simulink model "planner_contral"  (R2023b)
settings: Solver=FixedStepAuto  StartTime=0  StopTime=inf  FixedStep=0.001  RelTol=1e-3
undefined symbols (not defined in the file): aubr, c_factor, cf, cr, iniObsHeading1, iniObsHeading2, iniObsPos1, iniObsPos2, KD_PID_distance, KD_PID_speed, KI_PID_distance, KI_PID_speed, KP_PID_distance, KP_PID_speed, la, lb, LQR_K1, LQR_K2, LQR_K3, LQR_K4, m, rack_displacement, refInfo_obs1, refInfo_obs2, right_wheel_ground, rightWaypoints, tablebr, vubr, vx_break_point
libraries: Solver_SF x1
(part 6 of 8)

== matlab function planner_contral/decision_planning/EMplanner/spee planning with quadratic programming (qp) ==
  data: plan_start_s_dot input; qp_s_init output; plan_start_s_dot2 input; dp_speed_s input; dp_speed_t input; s_lb input; s_ub input; s_dot_lb input; s_dot_ub input; qp_s_dot_init output; qp_s_dot2_init output; relative_time_init output; w_cost_s_dot2 input; w_cost_v_ref input; w_cost_jerk input; w_ref_s input; speed_reference input
function [qp_s_init,qp_s_dot_init,qp_s_dot2_init,relative_time_init] = fcn(plan_start_s_dot,...
    plan_start_s_dot2,dp_speed_s,dp_speed_t,s_lb,s_ub,s_dot_lb,s_dot_ub,w_cost_s_dot2,w_cost_v_ref,w_cost_jerk,w_ref_s,speed_reference)

% 融合有限松弛约束的 QP 速度优化
% 原变量：每个节点 [s, s_dot, s_dot2]
% 新增变量：每个非起点节点 eps_s，用于轻微放松 s_lb / s_ub
%
% 松弛形式：
%   s >= s_lb - eps_s
%   s <= s_ub + eps_s
%   0 <= eps_s <= eps_s_max
%
% 注意：eps_s 惩罚权重较大，因此只有在原始边界接近不可行时才会启用

coder.extrinsic("solve_quadprog_safe");

% ---------- 参数 ----------
n = 17;
max_qp_node = 17;
default_speed_ub = 30;
large_s_bound = 1e4;

% 松弛变量参数
eps_s_max = 0.5;      % 最大允许纵向边界松弛量，单位 m
w_slack_s = 1e4;      % 松弛变量惩罚权重，越大越不愿意使用松弛

% ---------- 输出初始化 ----------
qp_s_init = ones(n,1) * nan;
qp_s_dot_init = ones(n,1) * nan;
qp_s_dot2_init = ones(n,1) * nan;
relative_time_init = ones(n,1) * nan;

% ---------- 计算有效 DP 点数 ----------
dp_speed_end = 16;
for i = 1:length(dp_speed_s)
    if isnan(dp_speed_s(i))
        dp_speed_end = i - 1;
        break;
    end
end

% DP 无有效点时，直接保守输出起点
if dp_speed_end < 1
    qp_s_init(1) = 0;
    qp_s_dot_init(1) = plan_start_s_dot;
    qp_s_dot2_init(1) = plan_start_s_dot2;
    relative_time_init(1) = 0;
    return;
end

recommend_T = dp_speed_t(dp_speed_end);
if ~isfinite(recommend_T) || recommend_T <= 0
    recommend_T = 8.0;
end

qp_size = dp_speed_end + 1;
if qp_size > max_qp_node
    qp_size = max_qp_node;
    dp_speed_end = qp_size - 1;
end

dt = recommend_T / dp_speed_end;
if ~isfinite(dt) || dt <= 0
    dt = 0.5;
end

% 原始变量数量：[s, v, a] * qp_size
old_var_num = 3 * qp_size;

% 新增松弛变量数量：非起点节点 qp_size - 1
slack_num = qp_size - 1;

% 总变量数量
var_num = old_var_num + slack_num;

% eps_s 在 X 中的起始位置
eps_offset = old_var_num;

% ---------- 等式约束：运动学连续性 ----------
% 原形式仍然是 Aeq' * X == beq
Aeq = zeros(var_num, 2*qp_size - 2);
beq = zeros(2*qp_size - 2, 1);

A_sub = [1, 0;
         dt, 1;
         (1/3)*dt^2, (1/2)*dt;
         -1, 0;
         0, -1;
         (1/6)*dt^2, dt/2];

for i = 1:qp_size - 1
    Aeq(3*i-2:3*i+3, 2*i-1:2*i) = A_sub;
end

% ---------- 不等式约束 ----------
% 1. 不允许倒车：s_i - s_{i+1} <= 0
% 2. 松弛下边界：-s_i - eps_i <= -s_lb
% 3. 松弛上边界： s_i - eps_i <=  s_ub

ineq_num = (qp_size - 1) + 2 * (qp_size - 1);
A = zeros(ineq_num, var_num);
b = zeros(ineq_num, 1);

row = 0;

% 不允许 s 后退
for i = 1:qp_size - 1
    row = row + 1;
    A(row, 3*i - 2) = 1;
    A(row, 3*i + 1) = -1;
    b(row) = 0;
end

% s 边界松弛约束
for i = 2:qp_size
    s_idx = 3*i - 2;
    eps_idx = eps_offset + (i - 1);

    cur_lb = s_lb(i-1);
    cur_ub = s_ub(i-1);

    % 防止 NaN / Inf 进入 quadprog
    if ~isfinite(cur_lb)
        cur_lb = 0;
    end

    if ~isfinite(cur_ub)
        cur_ub = large_s_bound;
    end

    cur_lb = max(cur_lb, 0);

    if cur_ub <= cur_lb
        cur_ub = cur_lb + 0.5;
    end

    % s_i >= cur_lb - eps_i
    % 等价于 -s_i - eps_i <= -cur_lb
    row = row + 1;
    A(row, s_idx) = -1;
    A(row, eps_idx) = -1;
    b(row) = -cur_lb;

    % s_i <= cur_ub + eps_i
    % 等价于 s_i - eps_i <= cur_ub
    row = row + 1;
    A(row, s_idx) = 1;
    A(row, eps_idx) = -1;
    b(row) = cur_ub;
end

% ---------- 变量上下界 ----------
lb = -inf(var_num, 1);
ub = inf(var_num, 1);

% 起点硬约束
lb(1) = 0;
lb(2) = plan_start_s_dot;
lb(3) = plan_start_s_dot2;
ub(1) = lb(1);
ub(2) = lb(2);
ub(3) = lb(3);

% 非起点的速度、加速度约束
for i = 2:qp_size
    s_idx = 3*i - 2;
    v_idx = 3*i - 1;
    a_idx = 3*i;

    % s 的具体上下边界已经通过 A,b 加入，这里只给物理范围
    lb(s_idx) = 0;
    ub(s_idx) = large_s_bound;

    cur_v_lb = s_dot_lb(i-1);
    cur_v_ub = s_dot_ub(i-1);

    if ~isfinite(cur_v_lb)
        cur_v_lb = 0;
    end

    if ~isfinite(cur_v_ub)
        cur_v_ub = default_speed_ub;
    end

    cur_v_lb = max(cur_v_lb, 0);

    if cur_v_ub <= cur_v_lb
        cur_v_ub = cur_v_lb + 0.1;
    end

    lb(v_idx) = cur_v_lb;
    ub(v_idx) = cur_v_ub;

    % 加速度硬约束
    lb(a_idx) = -6;
    ub(a_idx) = 4;
end

% 松弛变量约束：0 <= eps_s <= eps_s_max
for i = 1:slack_num
    eps_idx = eps_offset + i;
    lb(eps_idx) = 0;
    ub(eps_idx) = eps_s_max;
end

% ---------- 构造目标函数 ----------
A_s_dot2 = zeros(old_var_num, old_var_num);
A_jerk = zeros(old_var_num, qp_size - 1);
A_ref = zeros(old_var_num, old_var_num);
A_ref_s = zeros(old_var_num, old_var_num);

A4_sub = [0; 0; 1; 0; 0; -1];

for i = 1:qp_size
    A_s_dot2(3*i, 3*i) = 1;
    A_ref(3*i-1, 3*i-1) = 1;
    A_ref_s(3*i-2, 3*i-2) = 1;
end

for i = 1:qp_size - 1
    A_jerk(3*i-2:3*i+3, i) = A4_sub;
end

H_old = w_cost_s_dot2 * (A_s_dot2 * A_s_dot2') ...
      + w_cost_jerk * (A_jerk * A_jerk') ...
      + w_cost_v_ref * (A_ref * A_ref') ...
      + w_ref_s * (A_ref_s * A_ref_s');

H_old = 2 * H_old;

H = zeros(var_num, var_num);
H(1:old_var_num, 1:old_var_num) = H_old;

% 松弛变量二次惩罚
for i = 1:slack_num
    eps_idx = eps_offset + i;
    H(eps_idx, eps_idx) = 2 * w_slack_s;
end

f = zeros(var_num, 1);

% 推荐速度代价
for i = 1:qp_size
    f(3*i-1) = -2 * w_cost_v_ref * speed_reference;
end

% DP 纵向位置参考代价
for i = 1:dp_speed_end
    f(3*i-2) = -2 * w_ref_s * dp_speed_s(i);
end

% ---------- 求解 QP ----------
X = zeros(var_num, 1);
qp_ok = false;

[X, qp_ok] = solve_quadprog_safe(H, f, A, b, Aeq', beq, lb, ub, var_num);



if ~qp_ok
    qp_s_init(1) = 0;
    qp_s_dot_init(1) = plan_start_s_dot;
    qp_s_dot2_init(1) = plan_start_s_dot2;
    relative_time_init(1) = 0;

    last_s = 0;
    last_v = plan_start_s_dot;

    for i = 2:qp_size
        cur_s = dp_speed_s(i-1);

        if ~isfinite(cur_s)
            cur_s = last_s + max(last_v, 0) * dt;
        end

        cur_s = max(cur_s, last_s);

        if i >= 3
            cur_v = (cur_s - last_s) / dt;
        else
            cur_v = plan_start_s_dot;
        end

        if ~isfinite(cur_v)
            cur_v = speed_reference;
        end

        cur_v = max(cur_v, 0);
        cur_v = min(cur_v, default_speed_ub);

        qp_s_init(i) = cur_s;
        qp_s_dot_init(i) = cur_v;
        qp_s_dot2_init(i) = 0;
        relative_time_init(i) = (i - 1) * dt;

        last_s = cur_s;
        last_v = cur_v;
    end

    return;
end

% ---------- 正常输出 ----------
for i = 1:qp_size
    qp_s_init(i) = X(3*i - 2);
    qp_s_dot_init(i) = X(3*i - 1);
    qp_s_dot2_init(i) = X(3*i);
    relative_time_init(i) = (i - 1) * dt;
end

end

== matlab function planner_contral/decision_planning/EMplanner/Cartesian2Frenet/MATLAB Function2 ==
  data: ax_set input; s_dot2_set output; ay_set input; proj_heading_set input; proj_kappa_set input; l_set input; s_dot_set input; dl_set input; l_dot2_set output; ddl_set output
function [s_dot2_set,l_dot2_set,ddl_set] = fcn(ax_set,ay_set,proj_heading_set,proj_kappa_set,l_set,s_dot_set,dl_set)
%由于不知道有多少个点需要做坐标转换，设一个最大值做缓冲
n = 128;
% 输出初始化
s_dot2_set = ones(n,1)*nan;
l_dot2_set = ones(n,1)*nan;
ddl_set = ones(n,1)*nan;

for i = 1:length(l_set)
    if isnan(l_set(i))
       break;
    end
    a_h = [ax_set(i);ay_set(i)];
    n_r = [-sin(proj_heading_set(i));cos(proj_heading_set(i))];
    t_r = [cos(proj_heading_set(i));sin(proj_heading_set(i))];
    %近似认为dkr/ds 为0 简化计算
    l_dot2_set(i) = a_h'*n_r - proj_kappa_set(i) * (1 - proj_kappa_set(i) * l_set(i)) * s_dot_set(i)^2;
    s_dot2_set(i) = (1/(1 - proj_kappa_set(i) * l_set(i)))* (a_h' * t_r + 2 * proj_kappa_set(i) * dl_set(i) * s_dot_set(i)^2);
    % 要考虑加速度为0的情况
    if (s_dot2_set(i) < 1e-6)
        ddl_set(i) = 0;
    else
        ddl_set(i) = (l_dot2_set(i) - dl_set(i)*s_dot2_set(i))/(s_dot_set(i)^2);
    end
end

== matlab function planner_contral/decision_planning/EMplanner/generate st graph ==
  data: static_obs_s input; static_obs_l input; static_obs_heading input; dynamic_obs_s_set input; dynamic_obs_l_set input; dynamic_obs_heaidng_set input; static_obs_st_s_lb_set output; tra_s input; tra_l input; tra_path_indexs input; static_obs_st_s_ub_set output; dynamic_obs_st_s_lb_set output; dynamic_obs_st_s_ub_set output; obs_st_t_lb_set output; obs_st_t_ub_set output; static_obs_st_t_lb_set output; static_obs_st_t_ub_set output; plan_s_dot input; plan_l input; plan_s input; dynamic_obs_s_dot input; dynamic_obs_st_t_lb_set output; dynamic_obs_st_t_ub_set output
%%
% ============================================================
% generate ST graph
% 改进点：
% 1) 静态障碍物在整个规划时域内生成固定 ST 占用带；
% 2) 动态障碍物按 obs_s_dot 在每个时间步预测位置，生成连续 ST 占用带；
% 3) 多个障碍物暂时采用保守合并：同一时刻取最小 lb 和最大 ub；
% 4) 输入输出接口保持不变，便于直接替换原 Simulink MATLAB Function。
% ============================================================
function [static_obs_st_s_lb_set, static_obs_st_s_ub_set, ...
          dynamic_obs_st_s_lb_set, dynamic_obs_st_s_ub_set, ...
          obs_st_t_lb_set, obs_st_t_ub_set, ...
          static_obs_st_t_lb_set, static_obs_st_t_ub_set, ...
          dynamic_obs_st_t_lb_set, dynamic_obs_st_t_ub_set] = ...
    fcn(static_obs_s, static_obs_l, static_obs_heading, ...
        dynamic_obs_s_set, dynamic_obs_l_set, dynamic_obs_heaidng_set, ...
        tra_s, tra_l, tra_path_indexs, ...
        plan_s_dot, plan_l, plan_s, dynamic_obs_s_dot)

% -------- 基本参数 --------
n  = 81;
dt = 0.1;
t_grid = (0:dt:8)';

% -------- 初始化输出 --------
static_obs_st_s_lb_set  = ones(n,1) * inf;
static_obs_st_s_ub_set  = ones(n,1) * -inf;
dynamic_obs_st_s_lb_set = ones(n,1) * inf;
dynamic_obs_st_s_ub_set = ones(n,1) * -inf;

static_obs_st_t_lb_set  = t_grid;
static_obs_st_t_ub_set  = t_grid;
dynamic_obs_st_t_lb_set = t_grid;
dynamic_obs_st_t_ub_set = t_grid;

obs_st_t_lb_set = t_grid;
obs_st_t_ub_set = t_grid;

% -------- 静态障碍物 ST 边界 --------
[static_lb, static_ub] = getStaticBoundFullHorizon( ...
    static_obs_s, static_obs_l, static_obs_heading, ...
    tra_s, tra_l, tra_path_indexs, n, dt, plan_l, plan_s);

static_obs_st_s_lb_set = static_lb;
static_obs_st_s_ub_set = static_ub;

% -------- 动态障碍物 ST 边界 --------
[dynamic_lb, dynamic_ub] = getDynamicBoundFullHorizon( ...
    dynamic_obs_s_set, dynamic_obs_l_set, dynamic_obs_heaidng_set, ...
    tra_s, tra_l, tra_path_indexs, n, dt, plan_l, plan_s, dynamic_obs_s_dot);

dynamic_obs_st_s_lb_set = dynamic_lb;
dynamic_obs_st_s_ub_set = dynamic_ub;

end

%%
% ============================================================
% 静态障碍物：整个规划时域内保持固定 s/l/heading
% ============================================================
function [static_obs_lb, static_obs_ub] = getStaticBoundFullHorizon( ...
    static_obs_s, static_obs_l, static_obs_heading, ...
    tra_s, tra_l, index2s, n, dt, plan_l, plan_s)

vehLength = 5;
vehWidth  = 2;
vehHalfWidth = vehWidth / 2;

latThreshold = 2.7;

safeFront = 0;
safeRear  = 0;

startIgnoreDist = 3.0;

static_obs_lb = ones(n,1) * inf;
static_obs_ub = ones(n,1) * -inf;

% 当前接口只输出一组静态障碍物边界，
% 因此先选择当前规划路径上最近的一个前方障碍物。
best_lb = inf;
best_ub = -inf;
found = false;

for i = 1:length(static_obs_s)

    if isnan(static_obs_s(i))
        break;
    end

    rear_s = static_obs_s(i);
    rear_l = static_obs_l(i);
    heading = static_obs_heading(i);


    egoWidth = 2.0;
    latSafe = 0.2;
    lonSafe = 0.5;

    if ~isObstacleOverlapPathCorridor(rear_s, rear_l, heading, ...
        tra_s, tra_l, vehLength, vehWidth, egoWidth, latSafe, lonSafe)
        continue;
    end

    [lb_temp, ub_temp, valid] = calcObstacleSBound( ...
        rear_s, rear_l, heading, ...
        vehLength, vehHalfWidth, ...
        tra_s, tra_l, index2s);

    if ~valid
        continue;
    end

    lb_temp = lb_temp - safeRear;
    ub_temp = ub_temp + safeFront;

    % 忽略明显在起点附近或后方的障碍物
    if ub_temp <= plan_s + startIgnoreDist
        continue;
    end

    if lb_temp < plan_s + startIgnoreDist
        lb_temp = plan_s + startIgnoreDist;
    end

    % 只选择最近的前方障碍物
    if lb_temp < best_lb
        best_lb = lb_temp;
        best_ub = ub_temp;
        found = true;
    end
end

if found
    for j = 1:n
        static_obs_lb(j) = best_lb;
        static_obs_ub(j) = best_ub;
    end
end

end

%%
% ============================================================
% 动态障碍物：每个时间步用 s = s0 + v*t 预测
% ============================================================
function [dynamic_obs_lb, dynamic_obs_ub] = getDynamicBoundFullHorizon( ...
    dynamic_obs_s, dynamic_obs_l, dynamic_obs_heading, ...
    tra_s, tra_l, index2s, n, dt, plan_l, plan_s, obs_s_dot)

vehLength = 5;
vehWidth  = 2;
vehHalfWidth = vehWidth / 2;

latThreshold = 2.7;

safeFront = 0;
safeRear  = 0;

startIgnoreDist = 3.0;

dynamic_obs_lb = ones(n,1) * inf;
dynamic_obs_ub = ones(n,1) * -inf;

for j = 1:n

    t = (j-1) * dt;

    best_lb = inf;
    best_ub = -inf;
    found = false;

    for i = 1:length(dynamic_obs_s)

        if isnan(dynamic_obs_s(i))
            break;
        end

        s0 = dynamic_obs_s(i);
        l0 = dynamic_obs_l(i);
        heading = dynamic_obs_heading(i);

        if length(obs_s_dot) >= i
            v_obs = obs_s_dot(i);
        else
            v_obs = 0;
        end

        rear_s = s0 + v_obs * t;
        rear_l = l0;
     
        egoWidth = 2.0;
        latSafe = 0.2;
        lonSafe = 0.5;

        if ~isObstacleOverlapPathCorridor(rear_s, rear_l, heading, ...
                tra_s, tra_l, vehLength, vehWidth, egoWidth, latSafe, lonSafe)
           continue;
        end

        [lb_temp, ub_temp, valid] = calcObstacleSBound( ...
            rear_s, rear_l, heading, ...
            vehLength, vehHalfWidth, ...
            tra_s, tra_l, index2s);

        if ~valid
            continue;
        end

        lb_temp = lb_temp - safeRear;
        ub_temp = ub_temp + safeFront;

        if ub_temp <= plan_s + startIgnoreDist
            continue;
        end

        if lb_temp < plan_s + startIgnoreDist
            lb_temp = plan_s + startIgnoreDist;
        end

        % 每个时间步只选择最近的前方动态障碍物
        if lb_temp < best_lb
            best_lb = lb_temp;
            best_ub = ub_temp;
            found = true;
        end
    end

    if found
        dynamic_obs_lb(j) = best_lb;
        dynamic_obs_ub(j) = best_ub;
    end
end

end

%%
% ============================================================
% 根据障碍物 rear_s/rear_l/heading 计算其在参考路径上的 s 占用范围
% ============================================================
function [s_lb, s_ub, valid] = calcObstacleSBound( ...
    rear_s, rear_l, heading, ...
    vehLength, vehHalfWidth, ...
    tra_s, tra_l, index2s)

valid = false;
s_lb = inf;
s_ub = -inf;

% 前端点
front_s = rear_s + vehLength * cos(heading);
front_l = rear_l + vehLength * sin(heading);

% 四个角点
VehPoints = zeros(4,2);

VehPoints(1,1) = rear_s  - vehHalfWidth * sin(heading);
VehPoints(1,2) = rear_l  + vehHalfWidth * cos(heading);

VehPoints(2,1) = front_s - vehHalfWidth * sin(heading);
VehPoints(2,2) = front_l + vehHalfWidth * cos(heading);

VehPoints(3,1) = front_s + vehHalfWidth * sin(heading);
VehPoints(3,2) = front_l - vehHalfWidth * cos(heading);

VehPoints(4,1) = rear_s  + vehHalfWidth * sin(heading);
VehPoints(4,2) = rear_l  - vehHalfWidth * cos(heading);

index_matrix = zeros(4,1);

for z = 1:4

    dist_min = inf;
    index_min = 0;

    for k = 1:length(tra_s)

        if isnan(tra_s(k))
            break;
        end

        dist_s = tra_s(k) - VehPoints(z,1);
        dist_l = tra_l(k) - VehPoints(z,2);
        dist_temp = sqrt(dist_s^2 + dist_l^2);

        if dist_temp < dist_min
            dist_min = dist_temp;
            index_min = k;
        end
    end

    if index_min <= 0
        return;
    end

    index_matrix(z) = index_min;
end

min_index = min(index_matrix);
max_index = max(index_matrix);

if min_index <= 0 || max_index <= 0
    return;
end

if min_index > length(index2s) || max_index > length(index2s)
    return;
end

s_lb = index2s(min_index);
s_ub = index2s(max_index);

if ~isfinite(s_lb) || ~isfinite(s_ub)
    return;
end

if s_ub < s_lb
    temp = s_lb;
    s_lb = s_ub;
    s_ub = temp;
end

valid = true;

end

%%
% 判断障碍物矩形是否与当前规划路径走廊重叠
% rear_s, rear_l: 障碍物后轴/后端中心在 Frenet-like 坐标下的位置
% heading: 障碍物相对于 s-l 坐标的航向角
% tra_s, tra_l: 路径规划 DP+QP 后的最终路径
% obsLength, obsWidth: 障碍物长度和宽度
% egoWidth: ego 车辆宽度
% latSafe: 横向安全裕度
% lonSafe: 纵向安全裕度
function is_conflict = isObstacleOverlapPathCorridor( ...
    rear_s, rear_l, heading, ...
    tra_s, tra_l, obsLength, obsWidth, egoWidth, latSafe, lonSafe)

is_conflict = false;

obsHalfWidth = obsWidth / 2;
egoHalfWidth = egoWidth / 2;

% 横向膨胀后的半宽：障碍物半宽 + ego 半宽 + 安全裕度
latBound = obsHalfWidth + egoHalfWidth + latSafe;

% 纵向膨胀范围
u_min = -lonSafe;
u_max = obsLength + lonSafe;

% 只检查障碍物附近的路径点，避免远处路径点干扰
s_min_check = rear_s - lonSafe - 2.0;
s_max_check = rear_s + obsLength + lonSafe + 2.0;

cos_h = cos(heading);
sin_h = sin(heading);

for k = 1:length(tra_s)

    if isnan(tra_s(k))
        break;
    end

    s_path = tra_s(k);
    l_path = tra_l(k);

    if s_path < s_min_check || s_path > s_max_check
        continue;
    end

    % 将路径点转换到障碍物局部坐标系
    ds = s_path - rear_s;
    dl = l_path - rear_l;

    % u: 沿障碍物车身方向
    % v: 垂直障碍物车身方向
    u =  ds * cos_h + dl * sin_h;
    v = -ds * sin_h + dl * cos_h;

    % 路径中心线进入“障碍物膨胀矩形”，则认为有冲突
    if u >= u_min && u <= u_max && abs(v) <= latBound
        is_conflict = true;
        return;
    end
end

end

== matlab function planner_contral/decision_planning/EMplanner/speed decision with dynamic planning(dp) ==
  data: static_obs_s_lb input; dp_speed_s output; static_obs_s_ub input; dynamic_obs_s_lb input; dynamic_obs_s_ub input; obs_st_t_lb input; obs_st_t_ub input; dp_speed_t output; reference_speed_unlimit input; w_cost_ref_speed input; w_cost_accel input; w_cost_obs input; plan_start_s_dot input
function [dp_speed_s,dp_speed_t] = fcn(static_obs_s_lb,static_obs_s_ub,dynamic_obs_s_lb,dynamic_obs_s_ub,obs_st_t_lb,obs_st_t_ub,reference_speed_unlimit...
    ,w_cost_ref_speed,w_cost_accel,w_cost_obs,plan_start_s_dot)
% 速度动态规划
% 时间从0到8开始规划，最多8秒
% s的范围从0开始到路径规划的path的总长度为止
% 为了减少算力 采用非均匀采样，s越小的越密，越大的越稀疏

s_list = [0:0.5:4.5,...
          5.5:1:14.5,...
          16:1.5:29.5,...
          32:2.5:54.5];
% t 采用均匀采样每 0.5s采样一个点
t_list = 0.5:0.5:8;
% 声明st代价矩阵，表示从起点开始到(i,j)点的最小代价为dp_st_cost(i,j)
% s 采样40个 t 采样 16个 一共是 40 * 16
dp_st_cost = ones(40,16) * inf; % 首先初始化为无穷大
% dp_st_s_dot，表示从起点开始到(i,j)点的最优路径的末速度
dp_st_s_dot = zeros(40,16);
% 需要一个矩阵保持最优路径的前一个节点方便回溯
% dp_st_node(i,j) 表示位置为(i,j)的节点中，最优的上一层节点的行号为dp_st_node(i,j)
dp_st_node = zeros(40,16);
% 计算从dp起点到第一列的cost
for i = 1:length(s_list)
    dp_st_cost(i,1) = CalcDpCost(0,0,i,1,static_obs_s_lb,static_obs_s_ub,obs_st_t_lb,obs_st_t_ub,...
    w_cost_ref_speed,reference_speed_unlimit,w_cost_accel,w_cost_obs,plan_start_s_dot,s_list,t_list,dp_st_s_dot)+...
     CalcDpCost(0,0,i,1,dynamic_obs_s_lb,dynamic_obs_s_ub,obs_st_t_lb,obs_st_t_ub,...
    w_cost_ref_speed,reference_speed_unlimit,w_cost_accel,w_cost_obs,plan_start_s_dot,s_list,t_list,dp_st_s_dot);
    % 计算第一列所有节点的的s_dot，并存储到dp_st_s_dot中
    % 第一列的前一个节点只有起点，起点的s t 都是0
    [s_end,t_end] = CalcSTCoordinate(i,1,s_list,t_list);
    dp_st_s_dot(i,1) = s_end / t_end;
end
% 动态规划主程序
for i = 2:length(t_list)
    % i 为列循环
    for j = 1:length(s_list)
        % j 为行循环
        % 当前行为 j 列为 i
        cur_row = j;
        cur_col = i;
        % 遍历前一列
        for k = 1:length(s_list)
            pre_row = k;
            pre_col = i - 1;
            % 计算边的代价 其中起点为pre_row,pre_col 终点为cur_row cur_col
            cost_temp = CalcDpCost(pre_row,pre_col,cur_row,cur_col,static_obs_s_lb,static_obs_s_ub,obs_st_t_lb,obs_st_t_ub,...
                w_cost_ref_speed,reference_speed_unlimit,w_cost_accel,w_cost_obs,...
                plan_start_s_dot,s_list,t_list,dp_st_s_dot)+ CalcDpCost(pre_row,pre_col,cur_row,cur_col,dynamic_obs_s_lb,dynamic_obs_s_ub,obs_st_t_lb,obs_st_t_ub,...
              w_cost_ref_speed,reference_speed_unlimit,w_cost_accel,w_cost_obs,...
                plan_start_s_dot,s_list,t_list,dp_st_s_dot);
            if cost_temp + dp_st_cost(pre_row,pre_col) < dp_st_cost(cur_row,cur_col)
                dp_st_cost(cur_row,cur_col) = cost_temp + dp_st_cost(pre_row,pre_col);
                % 计算最优的s_dot
                [s_start,t_start] = CalcSTCoordinate(pre_row,pre_col,s_list,t_list);
                [s_end,t_end] = CalcSTCoordinate(cur_row,cur_col,s_list,t_list);
                dp_st_s_dot(cur_row,cur_col) = (s_end - s_start) / (t_end - t_start);
                % 将最短路径的前一个节点的行号记录下来
                dp_st_node(cur_row,cur_col) = pre_row;
            end      
        end
    end
end
% 输出初始化
dp_speed_s = ones(length(t_list),1) * nan;
dp_speed_t = dp_speed_s;
% 找到dp_node_cost 上边界和右边界代价最小的节点
min_cost = inf;
min_row = inf;
min_col = inf;
for i = 1:length(s_list)
    % 遍历右边界
    if dp_st_cost(i,length(t_list)) <= min_cost
        min_cost = dp_st_cost(i,length(t_list));
        min_row = i;
        min_col = length(t_list);
    end
end

for j = 1:length(t_list)
    % 遍历上边界
    if dp_st_cost(1,j) <= min_cost
        min_cost = dp_st_cost(1,j);
        min_row = 1;
        min_col = j;
    end
end
% 这里要注意，虽然我们在t上每0.5s采样一个时间，采了16个点，但是min_col 未必等于16
% 也就是说动态规划的最优解的时间未必是8秒
% 所以我们动态规划最后的输出s t 不一定是写满
% 先把终点的ST输出出来
[dp_speed_s(min_col),dp_speed_t(min_col)] = CalcSTCoordinate(min_row,min_col,s_list,t_list);
% 反向回溯
while min_col ~= 1
    pre_row = dp_st_node(min_row,min_col);
    pre_col = min_col - 1;
    [dp_speed_s(pre_col),dp_speed_t(pre_col)] = CalcSTCoordinate(pre_row,pre_col,s_list,t_list);
    min_row = pre_row;
    min_col = pre_col;
end


end

function cost = CalcDpCost(row_start,col_start,row_end,col_end,obs_st_s_in_set,obs_st_s_out_set,obs_st_t_in_set,obs_st_t_out_set,...
    w_cost_ref_speed,reference_speed,w_cost_accel,w_cost_obs,plan_start_s_dot,s_list,t_list,dp_st_s_dot)
    % 该函数将计算链接两个节点之间边的代价
    % 输入：边的起点的行列号row_start,col_start 边的终点行列号row_end,col_end
          % 障碍物st信息obs_st_s_in_set,obs_st_s_out_set,obs_st_t_in_set,obs_st_t_out_set
          % 推荐速度代价权重w_cost_ref_speed,加速度代价权重w_cost_accel,障碍物代价权重w_cost_obs
          % 推荐速度reference_speed
          % 拼接起点的速度plan_start_s_dot
          % s_list,t_list 采样距离
          % dp_st_s_dot 用于计算加速度
    % 首先计算终点的st坐标
    [s_end,t_end] = CalcSTCoordinate(row_end,col_end,s_list,t_list);
    % 规定起点的行列号为0 
    if row_start == 0
        % 边的起点为dp的起点
        s_start = 0;
        t_start = 0;
        s_dot_start = plan_start_s_dot;
    else
        % 边的起点不是dp的起点
        [s_start,t_start] = CalcSTCoordinate(row_start,col_start,s_list,t_list);
        s_dot_start = dp_st_s_dot(row_start,col_start);
    end
    cur_s_dot = (s_end - s_start) / (t_end - t_start);
    cur_s_dot2 = (cur_s_dot - s_dot_start)/(t_end - t_start);
    % 计算推荐速度代价
    cost_ref_speed = w_cost_ref_speed * (cur_s_dot - reference_speed)^2;
    % 计算加速度代价，这里注意，加速度不能超过车辆动力学上下限
    if cur_s_dot2 < 4 && cur_s_dot2 > -6
        cost_accel = w_cost_accel * cur_s_dot2^2;
    else
        % 超过车辆动力学限制，代价会增大很多倍
        cost_accel = 100000 * w_cost_accel * cur_s_dot2^2;
    end
    cost_obs = CalcObsCost(s_start,t_start,s_end,t_end,obs_st_s_in_set,obs_st_s_out_set,obs_st_t_in_set,obs_st_t_out_set,w_cost_obs);
    cost = cost_obs + cost_accel + cost_ref_speed;
end

function obs_cost = CalcObsCost(s_start,t_start,s_end,t_end,obs_st_s_in_set,obs_st_s_out_set,obs_st_t_in_set,obs_st_t_out_set,w_cost_obs)
% 该函数将计算边的障碍物代价
% 输入：边的起点终点s_start,t_start,s_end,t_end
%       障碍物信息 obs_st_s_in_set,obs_st_s_out_set,obs_st_t_in_set,obs_st_t_out_set
%       障碍物代价权重w_cost_obs
% 输出：边的障碍物代价obs_cost
  % 输出初始化
  obs_cost = 0;
  % 采样点的个数
  n = 5;
  % 采样时间间隔
  dt = (t_end - t_start)/(n - 1);
  % 边的斜率
  k = (s_end - s_start)/(t_end - t_start);
  for i = 1:n
      % 计算采样点的坐标
      t = t_start + (i - 1) * dt;
      s = s_start + k * (i - 1) * dt;
      % 遍历所有障碍物
      for j = 1:length(obs_st_s_in_set)
          if isnan(obs_st_s_in_set(j))
              continue;
          end
          % 计算点到st线段的最短距离
          vector1 = [obs_st_s_in_set(j);obs_st_t_in_set(j)] - [s;t];
          vector2 = [obs_st_s_out_set(j);obs_st_t_out_set(j)] - [s;t];
          vector3 = vector2 - vector1;
          min_dis = 0;
          dis1 = sqrt(vector1'*vector1);
          dis2 = sqrt(vector2'*vector2);
          dis3 = abs(vector1(1)*vector3(2) - vector1(2)*vector3(1))/sqrt(vector3'*vector3);
          if (vector1'*vector3 > 0 && vector2'*vector3 > 0) || (vector1'*vector3 < 0 && vector2'*vector3 < 0)
              min_dis = min(dis1,dis2);
          else
              min_dis = dis3;
          end
          obs_cost = obs_cost + CalcCollisionCost(w_cost_obs,min_dis); 
      end
  end
      
end

function collision_cost = CalcCollisionCost(w_cost_obs,min_dis)
  if abs(min_dis) < 0.5
      collision_cost = w_cost_obs;
  elseif abs(min_dis) > 0.5 && abs(min_dis) < 1.5
      % min_dis = 0.5    collision_cost = w_cost_obs^1;
      % min_dis = 1.5    collision_cost = w_cost_obs^0 = 1
      collision_cost = w_cost_obs^((0.5 - min_dis) + 1);
  else
      collision_cost = 0;
  end
end

function [s_value,t_value] = CalcSTCoordinate(row,col,s_list,t_list)
% 该函数将计算矩阵节点的s t 坐标
% 输入 row col 节点在矩阵的行号和列号
%      s_list t_list 采样间隔表
% 输出：s_value t_value 节点的 s t坐标
% 矩阵的(1,1) 代表的是最左上角的元素 s 最大 t 最小
% * 。。。。。。。。
% * 。。。。。。。。
% * 。。。。。。。。
% * 。。。。。。。。
% *****************

% 首先取出矩阵的行数
m = length(s_list);
% 1 1 对应的是 s 的最大值 t 的最小值
s_value = s_list(m - row + 1);
t_value = t_list(col);
end

== matlab function planner_contral/decision_planning/EMplanner/increase st point count ==
  data: s_init input; s output; s_dot_init input; s_dot2_init input; relative_time_init input; s_dot output; s_dot2 output; relative_time output
function [s,s_dot,s_dot2,relative_time] = fcn(s_init,s_dot_init,s_dot2_init,relative_time_init)
%该函数将增密s s_dot s_dot2
% 为什么需要增密，因为控制的执行频率是规划的10倍，轨迹点如果不够密，必然会导致规划效果不好
% 但是若在速度二次规划中点取的太多，会导致二次规划的矩阵规模太大计算太慢
% 所以方法是在二次规划中选取少量的点优化完毕后，在用此函数增密
t_end = length(relative_time_init);
for i = 1:length(relative_time_init)
    if isnan(relative_time_init(i))
        t_end = i - 1;
        break;
    end
end
T = relative_time_init(t_end);
n = 401;
dt = T/(n-1);
s = zeros(n,1);
s_dot = zeros(n,1);
s_dot2 = zeros(n,1);
relative_time = zeros(n,1);
for i = 1:n
    current_t = (i-1)*dt;
    for j = 1:t_end - 1
        if relative_time_init(j) <= current_t && relative_time_init(j+1) > current_t
            break;
        end
    end
    x = current_t - relative_time_init(j);
    s(i) = s_init(j) + s_dot_init(j)*x + (1/3)*s_dot2_init(j)*x^2 + (1/6)*s_dot2_init(j+1)*x^2; 
    s_dot(i) = s_dot_init(j) + 0.5*s_dot2_init(j)*x + 0.5*s_dot2_init(j+1)*x;
    s_dot2(i) = s_dot2_init(j) + (s_dot2_init(j+1) - s_dot2_init(j))*x/(relative_time_init(j+1) - relative_time_init(j));
    relative_time(i) = current_t;
end

== matlab function planner_contral/decision_planning/EMplanner/path and speed merge ==
  data: s input; trajectory_x output; s_dot input; s_dot2 input; relative_time input; current_time input; path_s input; trajectory_x_init input; trajectory_y_init input; trajectory_heading_init input; trajectory_kappa_init input; trajectory_y output; trajectory_heading output; trajectory_kappa output; trajectory_speed output; trajectory_accel output; trajectory_time output
function [trajectory_x,trajectory_y,trajectory_heading,trajectory_kappa,trajectory_speed,trajectory_accel,trajectory_time] = ...
    fcn(s,s_dot,s_dot2,relative_time,current_time,path_s,trajectory_x_init,trajectory_y_init,trajectory_heading_init,trajectory_kappa_init)
% 该函数将合并path和speed
% 由于path 是 60个点，speed 有 401个点，合并后，path和speed有401个点，因此需要做插值
n = 401;
trajectory_x = zeros(n,1);
trajectory_y = zeros(n,1);
trajectory_heading = zeros(n,1);
trajectory_kappa = zeros(n,1);
trajectory_speed = zeros(n,1);

trajectory_accel = zeros(n,1);
index = 1;
% 由于trajectory_x_init中不是所有的值都有效，(有nan) 所以要找到有效值的范围
while ~isnan(trajectory_x_init(index)) 
    index = index + 1;
end
index = index - 1;
trajectory_time = zeros(n,1);
for i = 1:n-1
    %interp1 线性插值
    % 若 x = [1,2] y = [3,4]
    %interp1(x,y,1.5) 会得到3.5
    %interp1 的缺点是 在端点或超过端点的，结果为nan
    % interp1(x,y,2) 不会等于4 而是会等于nan
    % interp1(x,y,6) 也会等于nan，所以在端点处要单独处理
    trajectory_x(i) = interp1(path_s(1:index),trajectory_x_init(1:index),s(i));
    trajectory_y(i) = interp1(path_s(1:index),trajectory_y_init(1:index),s(i));
    trajectory_heading(i) = interp1(path_s(1:index),trajectory_heading_init(1:index),s(i));
    trajectory_kappa(i) = interp1(path_s(1:index),trajectory_kappa_init(1:index),s(i));
    trajectory_time(i) = relative_time(i) + current_time;%速度规划会得到相对时间，转换成绝对时间
    trajectory_speed(i) = s_dot(i);
    trajectory_accel(i) = s_dot2(i);
end
% 端点单独处理
trajectory_x(end) = trajectory_x_init(end);
trajectory_y(end) = trajectory_y_init(end);
trajectory_heading(end) = trajectory_heading_init(end);
trajectory_kappa(end) = trajectory_kappa_init(end);
trajectory_time(end) = relative_time(end) + current_time;
trajectory_speed(end) = s_dot(end);
trajectory_accel(end) = s_dot2(end);

== matlab function planner_contral/decision_planning/EMplanner/stitch trajectory ==
  data: trajectory_x input; trajectory_x_final output; trajectory_y input; trajectory_heading input; trajectory_kappa input; trajectory_speed input; trajectory_accel input; trajectory_time input; stitch_x input; stitch_y input; stitch_heading input; stitch_kappa input; stitch_speed input; stitch_accel input; stitch_time input; trajectory_y_final output; trajectory_heading_final output; trajectory_kappa_final output; trajectory_speed_final output; trajectory_accel_final output; trajectory_time_final output
function [trajectory_x_final,trajectory_y_final,trajectory_heading_final,trajectory_kappa_final,...
          trajectory_speed_final,trajectory_accel_final,trajectory_time_final] = fcn(trajectory_x,...
          trajectory_y,trajectory_heading,trajectory_kappa,trajectory_speed,trajectory_accel,trajectory_time,...
          stitch_x,stitch_y,stitch_heading,stitch_kappa,stitch_speed,stitch_accel,stitch_time)
% 轨迹拼接，把stitch trajectory 拼到规划完成的轨迹上
n = 401 + 20;
trajectory_x_final = zeros(n,1);
trajectory_y_final = zeros(n,1);
trajectory_heading_final = zeros(n,1);
trajectory_kappa_final = zeros(n,1);
trajectory_speed_final = zeros(n,1);
trajectory_accel_final = zeros(n,1);
trajectory_time_final = zeros(n,1);

trajectory_x_final = [stitch_x;trajectory_x];
trajectory_y_final = [stitch_y;trajectory_y];
trajectory_heading_final = [stitch_heading;trajectory_heading];
trajectory_kappa_final = [stitch_kappa;trajectory_kappa];
trajectory_speed_final = [stitch_speed;trajectory_speed];
trajectory_accel_final = [stitch_accel;trajectory_accel];
trajectory_time_final = [stitch_time;trajectory_time];

== matlab function planner_contral/decision_planning/Visual/MATLAB Function ==
  data: static_s_lb input; static_s_ub input; dynamic_s_lb input; dynamic_s_ub input; dp_speed_s input; dp_speed_t input; qp_s_init input; t_time input; obs_st_t_lb_set input; obs_st_t_ub_set input; static_obs_st_t_lb_set input; static_obs_st_t_ub_set input; dynamic_obs_st_t_lb_set input; dynamic_obs_st_t_ub_set input; s_lb input; s_ub input
function visualization(static_s_lb,static_s_ub,dynamic_s_lb,dynamic_s_ub,dp_speed_s,dp_speed_t,qp_s_init,t_time,obs_st_t_lb_set,obs_st_t_ub_set,static_obs_st_t_lb_set,static_obs_st_t_ub_set,dynamic_obs_st_t_lb_set,dynamic_obs_st_t_ub_set, ...
    s_lb,s_ub)
%% 免编译声明
coder.extrinsic('fill');
coder.extrinsic('drivingScenario');
coder.extrinsic('laneMarking');
coder.extrinsic('lanespec');
coder.extrinsic('road');
coder.extrinsic('vehicle');
coder.extrinsic('advance');
coder.extrinsic('trajectory');
coder.extrinsic('findobj');
coder.extrinsic('delete');

%% ST图及DP、QP曲线
static_obsZone = zeros(162,2);

dynaimc_obsZone= zeros(162,2);



%%
num1 = 0;
num2 = 0;
for i = 1:81
     t = (i-1)*0.1;
    if ~isinf(static_s_lb(i))
        num1 = num1 + 1;
        static_obsZone(num1,:) = [t,static_s_lb(i)];
    end
   
    if ~isinf(dynamic_s_lb(i))
        num2 = num2 + 1;
        dynaimc_obsZone(num2,:) = [t,dynamic_s_lb(i)];
    end
end
% num3=0;
% num4=0;
% 上边界
for i =81:-1:1
     t = (i-1)*0.1;
    if ~isinf(static_s_ub(i))
        num1 = num1 + 1;
        static_obsZone(num1,:) = [t,static_s_ub(i)];
    end
    
    if ~isinf(dynamic_s_ub(i))
        num2 = num2+ 1;
        dynaimc_obsZone(num2,:) = [t,dynamic_s_ub(i)];
    end
end

figure(2)
clf
fill(static_obsZone(1:num1,1) ,static_obsZone(1:num1,2), 'b')
hold on
fill(dynaimc_obsZone(1:num2,1), dynaimc_obsZone(1:num2,2), 'b')
plot(dp_speed_t,dp_speed_s,'g-*');
hold on
plot(dp_speed_t,s_lb,'red-*');
hold on
plot(dp_speed_t,s_ub,'red-*');
plot(t_time,qp_s_init,'cyan-*');
grid on
xlim([0,8]);
ylim([0,60]);
xlabel('time / s')
ylabel('s/ m')

== stateflow chart planner_contral/Chart ==
  note: 规划-控制 频率解耦调度器
  note: ?
  note: 规划计数器i
  note: 控制计数器j
  (default) -> (junction 5)
  (junction 5) -> (junction 7)
  (junction 7) -> (junction 9) [order 1] : [i >= 100]
  (junction 7) -> (junction 13) [order 2] : {
      | i = i + 1;
      | }
  (junction 9) -> (junction 11) : {
      | do_planning;
      | i = 1;
      | }
  (junction 11) -> (junction 13)
  (junction 13) -> (junction 16)
  (junction 16) -> (junction 18) [order 1] : [j >= 10]
  (junction 16) -> (junction 22) [order 2] : {
      | j = j + 1;
      | }
  (junction 18) -> (junction 20) : {
      | do_control;
      | j = 1;
      | }
  (junction 20) -> (junction 22)
  (junction 22) -> (junction 25)
  data: i local =1; j local =1
  events: do_planning output FUNCTION_CALL_EVENT; do_control output FUNCTION_CALL_EVENT

== matlab function planner_contral/decision_planning/Visual/plot ==
  data: dp_s input; dp_l input; qp_s input; qp_l input; l_min input; l_max input; obs_s_set input; obs_l_set input; start_s input; start_l input; start_dl input; dynamic_s input; dynamic_l input; static_s_lb input; static_s_ub input; dynamic_s_lb input; dynamic_s_ub input
function  fcn(dp_s,dp_l,qp_s,qp_l,l_min,l_max,obs_s_set,obs_l_set,start_s,start_l,start_dl,dynamic_s,dynamic_l,static_s_lb,static_s_ub,dynamic_s_lb,dynamic_s_ub)
coder.extrinsic("plot","axis","figure","drawnow","cla","fill",'legend','set');
%该函数产生一个SL图
% 蓝线：dp_s, dp_l，DP 粗解轨迹
% 红线：qp_s, qp_l，QP 平滑/优化后的轨迹 动态规划粗轨迹 和 二次规划精轨迹
figure(1)
obs_length = 5;
obs_width = 2;
host_l = 5;
host_w = 1.6;
cla;
host_p1_l = start_l + sin(atan(start_dl)) * host_l /2 + host_w/2 * cos(atan(start_dl));
host_p1_s = start_s + cos(atan(start_dl)) * host_l /2 - host_w/2 * sin(atan(start_dl));
host_p2_l = start_l + sin(atan(start_dl)) * host_l /2 - host_w/2 * cos(atan(start_dl));
host_p2_s = start_s + cos(atan(start_dl)) * host_l /2 + host_w/2 * sin(atan(start_dl));
host_p3_l = start_l - sin(atan(start_dl)) * host_l /2 + host_w/2 * cos(atan(start_dl));
host_p3_s = start_s - cos(atan(start_dl)) * host_l /2 - host_w/2 * sin(atan(start_dl));
host_p4_l = start_l - sin(atan(start_dl)) * host_l /2 - host_w/2 * cos(atan(start_dl));
host_p4_s = start_s - cos(atan(start_dl)) * host_l /2 + host_w/2 * sin(atan(start_dl));
host_area_x = [host_p1_s;host_p2_s;host_p4_s;host_p3_s];
host_area_y = [host_p1_l;host_p2_l;host_p4_l;host_p3_l];
fill(host_area_x,host_area_y,'red');
hold on
h1=plot(dp_s,dp_l,'b');
h2=plot(qp_s,qp_l,'r');
% h3=plot(dp_s,l_min,'green');
%  h4= plot (dp_s,l_max,'green');
%   h = legend([h1 h3,h2,h4],'DP轨迹规划曲线','QP轨迹规划曲线','约束下边界','约束下边界');
%  set(h,'Fontname', 'Times New Roman','FontWeight','normal','FontSize',10,'linewidth',3)%% 单独设置legend的字体和格式 和后面用了7point大小 此处就不用了
grid on
xlabel('s/ m')
ylabel('l/ m')
axis([-4 61 -8 8]);
m=0;
for i = 1:length(obs_s_set)
    if isnan(obs_s_set(i))
        break;
    end
    obs_p1_s = obs_s_set(i) + obs_length/2;
    obs_p1_l = obs_l_set(i) + obs_width/2;
    obs_p2_s = obs_s_set(i) + obs_length/2;
    obs_p2_l = obs_l_set(i) - obs_width/2;
    obs_p3_s = obs_s_set(i) - obs_length/2;
    obs_p3_l = obs_l_set(i) + obs_width/2;
    obs_p4_s = obs_s_set(i) - obs_length/2;
    obs_p4_l = obs_l_set(i) - obs_width/2;
    obs_area_s = [obs_p1_s;obs_p2_s;obs_p4_s;obs_p3_s];
    obs_area_l = [obs_p1_l;obs_p2_l;obs_p4_l;obs_p3_l];
    fill(obs_area_s,obs_area_l,'blue');
end
for j=1:length(dynamic_s)
    if isnan(dynamic_s(j))
        continue;
    else
        m=m+1;
    end
end
a=1;
    dynamic_obs_p1_s = dynamic_s(a) + obs_length/2;
    dynamic_obs_p1_l =  dynamic_l(a) + obs_width/2;
    dynamic_obs_p2_s =dynamic_s(a) + obs_length/2;
    dynamic_obs_p2_l =dynamic_l(a) - obs_width/2;
    dynamic_obs_p3_s = dynamic_s(a) - obs_length/2;
    dynamic_obs_p3_l = dynamic_l(a) + obs_width/2;
    dynamic_obs_p4_s =  dynamic_s(a) - obs_length/2;
    dynamic_obs_p4_l = dynamic_l(a) - obs_width/2;
    dynamic_obs_area_s = [dynamic_obs_p1_s;dynamic_obs_p2_s;dynamic_obs_p4_s;dynamic_obs_p3_s];
    dynamic_obs_area_l = [dynamic_obs_p1_l;dynamic_obs_p2_l;dynamic_obs_p4_l;dynamic_obs_p3_l];
    fill(dynamic_obs_area_s,dynamic_obs_area_l,'blue');
  plot(dynamic_s(a:m),dynamic_l(a:m),'green')

end

== matlab function planner_contral/decision_planning/EMplanner/calc path length and map between point and s ==
  data: trajectory_x input; path_s_end output; trajectory_y input; path_s output
function [path_s_end,path_s] = fcn(trajectory_x,trajectory_y)
% 该函数将计算以trajectory的s 与 x y 的对应关系，可以看作是trajectory index2s
n = length(trajectory_x);
path_s = zeros(n,1);
sum = 0;
for i = 2:length(trajectory_x)
    if isnan(trajectory_x(i))
        break;
    end
    sum = sum + sqrt((trajectory_x(i) - trajectory_x(i-1))^2 + (trajectory_y(i) - trajectory_y(i-1))^2);
    path_s(i) = sum;
end
% 计算出trajectory的长度
if i == n
    path_s_end = path_s(end);
else
    % 因为循环的退出条件为isnan(trajectory_x(i)) 所以 i 所对应的数为 nan 
    path_s_end = path_s(i - 1);
end

== matlab function planner_contral/decision_planning/referenceline provider/reference_line_extraction ==
  data: host_match_point_index input; referenceline_x_init output; global_path_x input; global_path_y input; referenceline_y_init output
function [referenceline_x_init,referenceline_y_init] = fcn(host_match_point_index,global_path_x,global_path_y)
%该函数将在全局路径上提取referenceline的未平滑的初值
%输入： host_match_point_index 自车的位置在全局路径的匹配点的编号
       %global_path_x,global_path_y 全局路径数据
%输出：referenceline_x_init,referenceline_y_init 未平滑的参考线的xy坐标

%由于global path 是每1m取一个点，所以从匹配点往后取30个点，往前取150个点即可，一共181个点
%后面的点不够的话就用前面的点补，前面的点不够的话就用后面的点补，保证总数是181个

%索引初始化
start_index = -1;
%判断后面前面的点是否足够多
if host_match_point_index - 30 < 1
    %匹配点后面的点太少了，不够30个
    start_index = 1;
elseif host_match_point_index + 90 > length(global_path_x)
    %匹配点前面的点太少了，不够150个
    start_index = length(global_path_x) - 120;
    
else
    %匹配点正常情况
    start_index = host_match_point_index - 30;
end
%提取referenceline
referenceline_x_init = global_path_x(start_index:start_index + 120);
referenceline_y_init = global_path_y(start_index:start_index + 120);

== matlab function planner_contral/control module/MATLAB Function ==
  data: trajectory_x input; xr output; trajectory_y input; trajectory_heading input; trajectory_kappa input; trajectory_speed input; trajectory_accel input; trajectory_time input; current_time input; yr output; thetar output; kappar output; vr output; ar output
function [xr,yr,thetar,kappar,vr,ar] = fcn(trajectory_x,trajectory_y,trajectory_heading,...
    trajectory_kappa,trajectory_speed,trajectory_accel,trajectory_time,current_time)
% 该函数根据规划的轨迹计算出期望跟踪的点
% 由于控制也是有延迟，所以控制发出的期望跟踪的点是current_time + 0.01;
control_time = current_time + 0.01;
% 规划发出的轨迹有一部分是拼接的，在刚启动的时候，stitch_time = -1,因此要先把它去掉
start_index = 1;
while (trajectory_time(start_index) == -1)
    start_index = start_index + 1;
end
% 使用interp1插值计算得到xr yr thetar,kappar,vr,ar
% 由于interp1在端点会得到nan，因此需要防一手
% 解释，为什么需要trajectory_time(start_index) ~= 0
% 因为在刚启动时规划先执行(100ms)，当规划完毕的时候控制已经执行了10次
% 那么在最开始的时候，规划还没给结果是控制已经执行了10次，在这10次中控制跟踪的轨迹是空轨迹
% simulink 空轨迹表示为 0，0，0，0，0，0......,这样trajectory_time
% 也全是0，trajectory_time不单调递增
% 而interp1(x,y,x0)要求x必须要单调递增，否则会报错，所以当规划首次运行时控制需要执行下面这个else分支的代码，否则会报错
if control_time > trajectory_time(start_index) && trajectory_time(start_index) ~= 0
    xr = interp1(trajectory_time(start_index:end),trajectory_x(start_index:end),control_time);
    yr = interp1(trajectory_time(start_index:end),trajectory_y(start_index:end),control_time);
    thetar = interp1(trajectory_time(start_index:end),trajectory_heading(start_index:end),control_time);
    kappar = interp1(trajectory_time(start_index:end),trajectory_kappa(start_index:end),control_time);
    vr = interp1(trajectory_time(start_index:end),trajectory_speed(start_index:end),control_time);
    ar = interp1(trajectory_time(start_index:end),trajectory_accel(start_index:end),control_time);
else
    xr = trajectory_x(start_index);
    yr = trajectory_y(start_index);
    thetar = trajectory_heading(start_index);
    kappar = trajectory_kappa(start_index);
    vr = trajectory_speed(start_index);
    ar = trajectory_accel(start_index);
end

== matlab function planner_contral/control module/control main/chassic steering system/MATLAB Function ==
  data: u input; right_steer output; la input; lb input
function right_steer = fcn(u,la,lb)
if abs(u)<1e-2
   right_steer = u;
else
   R =  (la+lb)/tan(u);
   right_steer = atan((la+lb)/(R+1.624/2));
end

== matlab function planner_contral/decision_planning/referenceline provider/calculate heading&kappa 2 ==
  data: path_x input; path_heading output; path_y input; path_kappa output
function [path_heading,path_kappa] = fcn(path_x,path_y)
%该函数将计算path的切线方向与x轴的夹角和曲率
%输入：path_x,y路径坐标
%输出：path heading kappa 路径的heading和曲率
%原理 heading = arctan(dy/dx);
%     kappa = dheading/ds;
%     ds = (dx^2 + dy^2)^0.5

%注意，角度的多值性会带来很大的麻烦，需要慎重处理
%例，x 与 x + 2pi往往代表同一个角度，这种多值性在计算曲率会带来麻烦
%比如 原本是(0.1 - (-0.1))/ds，但如果计算出的-0.1多了一个2pi
%kappa就等于(0.1 - (-0.1 + 2*pi))/ds，曲率会变得非常大
%还有若采用中点欧拉法计算heading时，(即使用(y2 - y1)/(x2 - x1)的反正切计算一个角度 ，用(y1 - y0)/(x1
%-x0)的反正切又计算一个角度，然后加起来除以2),如果精确值是 (a1 + a2)/2,但最终计算的结果可能是(a1 + a2 + 2pi)/2
% 还有 tan(x) = tan(x + pi) 所以arctan(tan(x))可能等于x，也可能等于x + pi
% 角度的处理非常麻烦，而且角度处理不当往往是许多奇怪错误的源头

dx = diff(path_x);
dy = diff(path_y);
%用中点欧拉法要比向前欧拉法向后欧拉法更精确，但是也可能计算出的结果比精确值多一个pi
%在这里对dx,dy做中点欧拉法，使用四象限反正切计算角度
dx_pre = [dx(1);dx];
dx_after = [dx;dx(end)];
dx_final = (dx_pre + dx_after)/2;

dy_pre = [dy(1);dy];
dy_after = [dy;dy(end)];
dy_final = (dy_pre + dy_after)/2;

ds_final = sqrt(dx_final.^2 + dy_final.^2);
path_heading = atan2(dy_final,dx_final);

dheading = diff(path_heading);
dheading_pre = [dheading(1);dheading];
dheading_after = [dheading;dheading(end)];
dheading_final = (dheading_pre + dheading_after) / 2;
%为了防止dheading出现多一个2pi的错误，假设真实的dheading较小，用sin(dheading)近似dheading
path_kappa = sin(dheading_final) ./ ds_final;

== matlab function planner_contral/decision_planning/referenceline provider/reference_line_smoothing ==
  data: referenceline_x_init input; referenceline_x output; referenceline_y_init input; w_cost_smooth input; w_cost_length input; w_cost_ref input; x_lb input; x_ub input; y_lb input; y_ub input; referenceline_y output
function [referenceline_x,referenceline_y] = ...
    fcn(referenceline_x_init,referenceline_y_init,w_cost_smooth,w_cost_length,w_cost_ref,x_lb,x_ub,y_lb,y_ub)
%该函数将平滑referenceline
%使用二次规划
%0.5x'Hx + f'x = min
% lb < x < ub
% 输入 referenceline x,y,init未平滑的参考线
% w_cost_smooth,w_cost_length,w_cost_ref 平滑代价，紧凑代价，几何相似代价权重系数
% x_lb,x_ub,y_lb,y_ub 允许x,y变化的上下界
% 输出 referenceline_x,referenceline_y 平滑后的参考线

%在这里为了简化，不使用参考线拼接算法
%计算量问题通过调度解决，规划周期为100ms，只要在100ms计算完就可以
%如果到最后计算速度成问题在优化，目前暂时不使用拼接

%simulink无法直接使用自带的二次规划函数，需要从外部引入

coder.extrinsic("quadprog");
% 二次规划形式
% H1 = w_cost_smooth*(A1'*A1) + w_cost_length*(A2'*A2) + w_cost_ref*(A3'*A3)
% f = -2 * w_cost_ref * referenceline_init
% x'H1x + f'x = 0.5 * x'(2H1)*x + f'x
% A1 = [1  0 -2  0  1  0
%       0  1  0 -2  0  1
%             1  0 -2  0  1  0
%             0  1  0 -2  0  1
%                   ...............
%A2 = [1  0 -1  0
%      0  1  0 -1
%            1  0 -1  0
%            0  1  0 -1
%                  ...........
%A3 为单位矩阵
%设置求解矩阵规模，因为参考线初始点一共181个，每个点有两个坐标，所以求解矩阵规模是362个
n = 121;
%referenceline初始化
referenceline_x = zeros(n,1);
referenceline_y = zeros(n,1);

A1 = zeros(2 * n - 4, 2 * n);
A2 = zeros(2 * n - 2, 2 * n);
A3 = eye(2 * n, 2 * n);
f = zeros(2 * n, 1);
lb = zeros(2 * n, 1);
ub = zeros(2 * n, 1);
persistent is_first_run;
persistent pre_result_x;
persistent pre_result_y;
persistent pre_referenceline_x_init;
persistent pre_referenceline_y_init;

if isempty(is_first_run)
    is_first_run = 0;
    for i = 1 : n
        f(2 * i - 1) = referenceline_x_init(i);
        f(2 * i) = referenceline_y_init(i);
        lb(2 * i - 1) = f(2 * i - 1) + x_lb;
        ub(2 * i - 1) = f(2 * i - 1) + x_ub;
        lb(2 * i) = f(2 * i) + y_lb;
        ub(2 * i) = f(2 * i) + y_ub;
    end

    for j = 1 : 2 * n - 5
        A1(j , j) = 1;
        A1(j , j + 2) = -2;
        A1(j , j + 4) = 1;
        A1(j + 1, j + 1) = 1;
        A1(j + 1, j + 3) = -2;
        A1(j + 1, j + 5) = 1;
    end

    for k = 1 : 2 * n - 3
        A2(k, k) = 1;
        A2(k, k + 2) = -1;
        A2(k + 1, k + 1) = 1;
        A2(k + 1, k + 3) = -1;
    end

    H1 = w_cost_smooth * (A1'*A1) + w_cost_length * (A2'*A2) + w_cost_ref * A3;
    H = 2 * H1;
    %用 referenceline 的初值作为二次规划的迭代起点
    X0 = f;
    f = -2 * w_cost_ref * f;
    %二次规划求解
    X = quadprog(H,f,[],[],[],[],lb,ub,X0);
    %将结果输出到referenceline中
    for i = 1 : n
        referenceline_x(i) = X(2 * i - 1);
        referenceline_y(i) = X(2 * i);
    end
    pre_result_x = referenceline_x;
    pre_result_y = referenceline_y;
    pre_referenceline_x_init = referenceline_x_init;
    pre_referenceline_y_init = referenceline_y_init;
else
    if pre_referenceline_x_init(1) == referenceline_x_init(1) && ...
            pre_referenceline_y_init(1) == referenceline_y_init(1)
        %起点相同，可以认为本周期和上周期的referenceline_init 一模一样，就直接复用上个周期的结果
        referenceline_x = pre_result_x;
        referenceline_y = pre_result_y;
    else
        %起点不同。重复第一次运行的逻辑
        for i = 1 : n
            f(2 * i - 1) = referenceline_x_init(i);
            f(2 * i) = referenceline_y_init(i);
            lb(2 * i - 1) = f(2 * i - 1) + x_lb;
            ub(2 * i - 1) = f(2 * i - 1) + x_ub;
            lb(2 * i) = f(2 * i) + y_lb;
            ub(2 * i) = f(2 * i) + y_ub;
        end

        for j = 1 : 2 * n - 5
            
            A1(j , j) = 1;
            A1(j , j + 2) = -2;
            A1(j , j + 4) = 1;
            A1(j + 1, j + 1) = 1;
            A1(j + 1, j + 3) = -2;
            A1(j + 1, j + 5) = 1;
        end

        for k = 1 : 2 * n - 3
            A2(k, k) = 1;
            A2(k, k + 2) = -1;
            A2(k + 1, k + 1) = 1;
            A2(k + 1, k + 3) = -1;
        end

        H1 = w_cost_smooth * (A1'*A1) + w_cost_length * (A2'*A2) + w_cost_ref * A3;
        H = 2 * H1;
        %用 referenceline 的初值作为二次规划的迭代起点
        X0 = f;
        f = -2 * w_cost_ref * f;
        %二次规划求解
        X = quadprog(H,f,[],[],[],[],lb,ub,X0);
        %将结果输出到referenceline中
        for i = 1 : n
            referenceline_x(i) = X(2 * i - 1);
            referenceline_y(i) = X(2 * i);
        end
        pre_result_x = referenceline_x;
        pre_result_y = referenceline_y;
        pre_referenceline_x_init = referenceline_x_init;
        pre_referenceline_y_init = referenceline_y_init;
        
    end
    
end
